simulink model "Modelo_Vibratorio_simulink"  (R2020a)
settings: Solver=ode15s  StartTime=0.0  StopTime=10.0  MaxStep=0.001  RelTol=1e-3
undefined symbols (not defined in the file): A, B, Cc, D, v0, x0
settings Model: Creator=Noxi-PC  LastModifiedBy=Noxi-PC

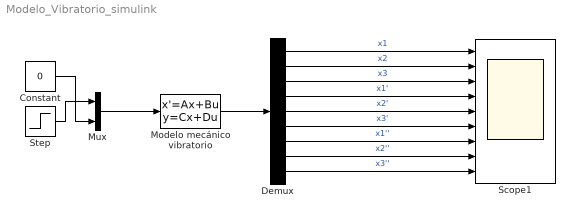
== system Modelo_Vibratorio_simulink ==
  Constant : Constant  Value=0
  Demux : Demux  Outputs=9
  Modelo mecánico vibratorio : StateSpace  A=A  B=B  C=Cc  D=D  InitialCondition=[x0,v0]
  Mux : Mux  Inputs=2
  Scope1 : Scope  NumInputPorts=9
  Step : Step  After=80  SampleTime=0
  wires:
  Modelo mecánico vibratorio/1 -> Demux/1
  Demux/1 -> Scope1/1  "x1"
  Demux/2 -> Scope1/2  "x2"
  Demux/3 -> Scope1/3  "x3"
  Demux/4 -> Scope1/4  "x1'"
  Demux/5 -> Scope1/5  "x2'"
  Demux/6 -> Scope1/6  "x3'"
  Demux/7 -> Scope1/7  "x1''"
  Demux/8 -> Scope1/8  "x2''"
  Demux/9 -> Scope1/9  "x3''"
  Mux/1 -> Modelo mecánico vibratorio/1
  Constant/1 -> Mux/2
  Step/1 -> Mux/1
